simulink model "Inner3"  (Simulink 5.0)
settings: Solver=ode45  StartTime=0.0  StopTime=10.0  RelTol=1e-3
undefined symbols (not defined in the file): sigbuilder_block
settings Model: Creator=scaife  LastModifiedBy=scaife  ExtModeAutoUpdateStatusClock=off

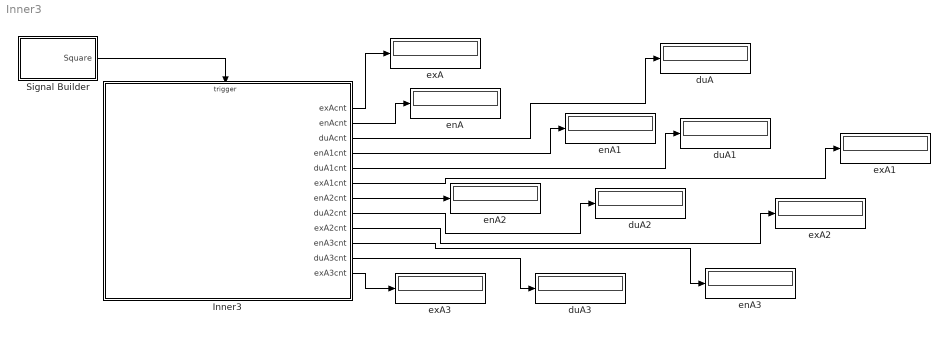
== system Inner3 ==
  Inner3 : Stateflow chart
  Signal Builder : Subsystem  Tag=STV Subsys  StartFcn=sigbuilder_block('start');  StopFcn=sigbuilder_block('stop');  ClipboardFcn=sigbuilder_block('clipboard');  mask(Sigbuilder block){}
      mask help: Sigbuilder GUI
      mask init:
      | if ~strcmp(get_param(bdroot(gcb),'SimulationStatus'),'stopped') tuvar = sigbuilder_block('maskInit'); end
      settings: CopyFcn=sigbuilder_block('copy');  DeleteFcn=sigbuilder_block('delete');  ModelCloseFcn=sigbuilder_block('modelClose');  PreSaveFcn=sigbuilder_block('preSave');  NameChangeFcn=sigbuilder_block('namechange');  OpenFcn=sigbuilder_block('open',[50 50 520 400 ]);  CloseFcn=sigbuilder_block('close');
      mask Display: plot(0,0,100,100,[10,10,40,40,10],[80,20,20,80,80],[40,10],[50,50], [40,27,10],[65,72,56],[40,25,25,10],[28,28,43,43]);
  duA{,1..3} (4 alike) : Display
  enA{,1..3} (4 alike) : Display
  exA{,1..3} (4 alike) : Display
  wires:
  Signal Builder/1(Square) -> Inner3/Trigger
  Inner3/1(exAcnt) -> exA/1
  Inner3/2(enAcnt) -> enA/1
  Inner3/3(duAcnt) -> duA/1
  Inner3/4(enA1cnt) -> enA1/1
  Inner3/5(duA1cnt) -> duA1/1
  Inner3/6(exA1cnt) -> exA1/1
  Inner3/7(enA2cnt) -> enA2/1
  Inner3/8(duA2cnt) -> duA2/1
  Inner3/9(exA2cnt) -> exA2/1
  Inner3/12(exA3cnt) -> exA3/1
  Inner3/11(duA3cnt) -> duA3/1
  Inner3/10(enA3cnt) -> enA3/1

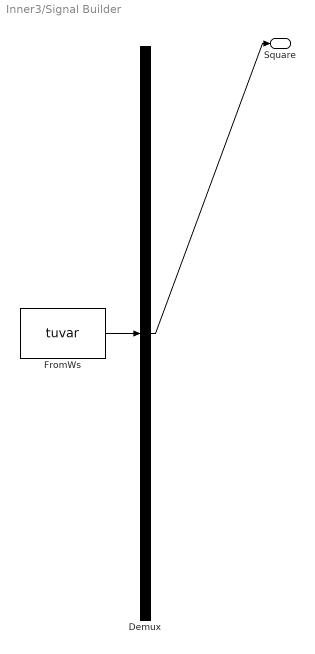
== system Inner3/Signal Builder ==
  Demux : Demux  Tag=STV Demux  Outputs=1
  FromWs : FromWorkspace  Tag=STV FromWs  VariableName=tuvar  SampleTime=0  SigBuilderData=DataTag0
  Square : Outport  Tag=STV Outport
  wires:
  FromWs/1 -> Demux/1
  Demux/1 -> Square/1

== stateflow chart Inner3 ==
  state A/
    en: enAcnt++;
    du: duAcnt++;
    ex: exAcnt++;
    state A1/
      en: enA1cnt++;
      du: duA1cnt++;
      ex: exA1cnt++;
    state A2/
      en: enA2cnt++;
      du: duA2cnt++;
      ex: exA2cnt++;
    state A3/
      en: enA3cnt++;
      du: duA3cnt++;
      ex: exA3cnt++;
    A -> (junction 7) : E
    (junction 7) -> A1 : [duAcnt%%3==0]
    (junction 7) -> A2 : [duAcnt%%3==1]
    (junction 7) -> A3 : [duAcnt%%3==2]
    (default) -> A1
  (default) -> A
  data: exAcnt output int32; enAcnt output int32; duAcnt output int32; enA1cnt output int32; duA1cnt output int32; exA1cnt output int32; enA2cnt output int32; duA2cnt output int32; exA2cnt output int32; enA3cnt output int32; duA3cnt output int32; exA3cnt output int32
  events: E input EITHER_EDGE_EVENT
